simulink model "InertialSimulink"  (R2017a)
settings: Solver=VariableStepAuto  StartTime=0.0  StopTime=18  RelTol=1e-3
values from neighbouring files (symbols this model uses):
  c1 = 11    [InertialMatlab.m]
  c2 = 5    [InertialMatlab.m]
  d1 = 0.2    [InertialMatlab.m]
  d2 = 1.0    (= 1)    [InertialMatlab.m]
  J1 = 0.4    [InertialMatlab.m]
  J2 = 1.0    (= 1)    [InertialMatlab.m]
libraries: simulink x1
settings Model: Creator=mortenmj  LastModifiedBy=mortenmj

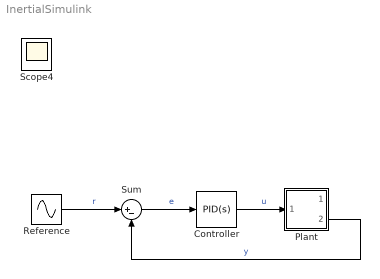
== system InertialSimulink ==
  Controller : simulink/Continuous/PID Controller  Controller=PID  TimeDomain=Continuous-time  SampleTime=-1  IntegratorMethod=Forward Euler  FilterMethod=Forward Euler  Form=Parallel  UseFilter=on  ControllerParametersSource=internal  P=1  I=1  D=0  N=100  InitialConditionSource=internal  InitialConditionForIntegrator=0  InitialConditionForFilter=0  ExternalReset=none  LimitOutput=off  UpperSaturationLimit=inf  LowerSaturationLimit=-inf  LinearizeAsGain=on  AntiWindupMode=none  Kb=1  TrackingMode=off  Kt=1  PParamMin=[]  PParamMax=[]  IParamMin=[]  IParamMax=[]  DParamMin=[]  DParamMax=[]  NParamMin=[]  NParamMax=[]  KbParamMin=[]  KbParamMax=[]  KtParamMin=[]  KtParamMax=[]  POutMin=[]  POutMax=[]  IOutMin=[]  IOutMax=[]  DOutMin=[]  DOutMax=[]  NOutMin=[]  NOutMax=[]  KbOutMin=[]  KbOutMax=[]  KtOutMin=[]  KtOutMax=[]  IntegratorOutMin=[]  IntegratorOutMax=[]  FilterOutMin=[]  FilterOutMax=[]  SumOutMin=[]  SumOutMax=[]  SumI1OutMin=[]  SumI1OutMax=[]  SumI2OutMin=[]  SumI2OutMax=[]  SumI3OutMin=[]  SumI3OutMax=[]  SumDOutMin=[]  SumDOutMax=[]  SaturationOutMin=[]  SaturationOutMax=[]  IntegratorContinuousStateAttributes=''  IntegratorStateMustResolveToSignalObject=off  IntegratorRTWStateStorageClass=Auto  FilterContinuousStateAttributes=''  FilterStateMustResolveToSignalObject=off  FilterRTWStateStorageClass=Auto  DifferentiatorICPrevScaledInput=0  DifferentiatorOutMin=[]  DifferentiatorOutMax=[]  InitialConditionSetting=State (most efficient)
  Plant : ModelReference  ModelNameDialog=Plant.slx  ParameterArgumentNames=J1,J2,c1,c2,d1,d2  ParameterArgumentValues=J1,J2,c1,c2,d1,d2  UsingDefaultArgumentValue=0,0,0,0,0,0  SimulationMode=Normal  ModelReferenceVersion=1.29  J1=J1  c1=c1  J2=J2  c2=c2  d1=d1  d2=d2
  Reference : Sin
  Sum : Sum  Inputs=|+-
  Scope4 : Scope
  wires:
  Reference/1 -> Sum/1  "r"
  Plant/2 -> Sum/2  "y"
  Controller/1 -> Plant/1  "u"
  Sum/1 -> Controller/1  "e"
